simulink model "sampleModel7126_pp"  (R2018a)
settings: Solver=VariableStepAuto  StartTime=0.0  StopTime=10.0  RelTol=1e-3
undefined symbols (not defined in the file or in its folder): DiscIntNeverNeededParam
libraries: simulink x367
(part 4 of 8)

== system sampleModel7126_pp/cfblk275 ==
  cfblk1 : Inport
  Action Port : ActionPort  ActionType=then
  cfblk10 : Subsystem  TreatAsAtomicUnit=on
  cfblk11 : Subsystem  TreatAsAtomicUnit=on
  cfblk12 : Delay
  cfblk13 : Delay
  cfblk3 : simulink/Discrete/Transfer Fcn Real Zero  ZeroZ=0.75  ICPrevInput=0.0  DoSatur=off
      settings: SourceProductName=Simulink  SourceProductBaseCode=SL
  cfblk4 : simulink/Discrete/Transfer Fcn Real Zero  ZeroZ=0.75  ICPrevInput=0.0  DoSatur=off
      settings: SourceProductName=Simulink  SourceProductBaseCode=SL
  cfblk5 : simulink/Continuous/PID Controller  Controller=PID  TimeDomain=Discrete-time  SampleTime=-1  IntegratorMethod=Forward Euler  FilterMethod=Forward Euler  Form=Parallel  UseFilter=on  ControllerParametersSource=internal  P=1  I=1  D=0  N=100  InitialConditionSource=internal  InitialConditionForIntegrator=0  InitialConditionForFilter=0  ExternalReset=none  LimitOutput=off  UpperSaturationLimit=inf  LowerSaturationLimit=-inf  LinearizeAsGain=off  AntiWindupMode=none  Kb=1  TrackingMode=off  Kt=1  PParamMin=[]  PParamMax=[]  IParamMin=[]  IParamMax=[]  DParamMin=[]  DParamMax=[]  NParamMin=[]  NParamMax=[]  KbParamMin=[]  KbParamMax=[]  KtParamMin=[]  KtParamMax=[]  POutMin=[]  POutMax=[]  IOutMin=[]  IOutMax=[]  DOutMin=[]  DOutMax=[]  NOutMin=[]  NOutMax=[]  KbOutMin=[]  KbOutMax=[]  KtOutMin=[]  KtOutMax=[]  IntegratorOutMin=[]  IntegratorOutMax=[]  FilterOutMin=[]  FilterOutMax=[]  SumOutMin=[]  SumOutMax=[]  SumI1OutMin=[]  SumI1OutMax=[]  SumI2OutMin=[]  SumI2OutMax=[]  SumI3OutMin=[]  SumI3OutMax=[]  SumDOutMin=[]  SumDOutMax=[]  SaturationOutMin=[]  SaturationOutMax=[]  IntegratorContinuousStateAttributes=''  IntegratorStateMustResolveToSignalObject=off  IntegratorRTWStateStorageClass=Auto  FilterContinuousStateAttributes=''  FilterStateMustResolveToSignalObject=off  FilterRTWStateStorageClass=Auto  DifferentiatorICPrevScaledInput=0  DifferentiatorOutMin=[]  DifferentiatorOutMax=[]  FilterDiffOutCoefMin=[]  FilterDiffOutCoefMax=[]  SumDenOutMin=[]  SumDenOutMax=[]  SumNumOutMin=[]  SumNumOutMax=[]  ReciprocalOutMin=[]  ReciprocalOutMax=[]  DivideOutMin=[]  DivideOutMax=[]  TunerSelectOption=Transfer Function Based (PID Tuner App)
  cfblk6 : simulink/Discrete/Difference  ICPrevInput=0.0  OutMin=[]  OutMax=[]  OutDataTypeStr=double  OutputDataTypeScalingMode=double  OutDataType=fixdt(1, 16)  OutScaling=2^-10  DoSatur=off
  cfblk7 : DiscreteStateSpace  SampleTime=-1
  cfblk8 : DiscreteIntegrator  SampleTime=-1  OutDataTypeStr=double  ICPrevOutput=DiscIntNeverNeededParam  ICPrevScaledInput=DiscIntNeverNeededParam
  cfblk9 : If  SampleTime=1
  cyemi_{764,777,792..800} (11 alike) : DataTypeConversion  OutDataTypeStr=double
  cfblk2 : Outport
  wires:
  cfblk1/1 -> cfblk2/1
  cfblk9/1 -> cfblk10/Action
  cfblk9/2 -> cfblk11/Action
  cyemi_764/1 -> cfblk10/1(cfblk1)
  cfblk11/2(cfblk15) -> cyemi_764/1
  cyemi_777/1 -> cfblk11/1(cfblk1)
  cfblk13/1 -> cyemi_777/1
  cyemi_792/1 -> cfblk12/1
  cfblk5/1 -> cyemi_792/1
  cyemi_793/1 -> cfblk13/1
  cfblk8/1 -> cyemi_793/1
  cyemi_794/1 -> cfblk3/1
  cfblk12/1 -> cyemi_794/1
  cyemi_795/1 -> cfblk4/1
  cfblk6/1 -> cyemi_795/1
  cyemi_796/1 -> cfblk5/1
  cfblk11/1(cfblk2) -> cyemi_796/1
  cyemi_797/1 -> cfblk6/1
  cfblk3/1 -> cyemi_797/1
  cyemi_798/1 -> cfblk7/1
  cfblk11/3(cfblk16) -> cyemi_798/1
  cyemi_799/1 -> cfblk8/1
  cfblk7/1 -> cyemi_799/1
  cyemi_800/1 -> cfblk9/1
  cfblk4/1 -> cyemi_800/1

== system sampleModel7126_pp/cfblk276 ==
  cfblk1 : Inport
  cfblk9 : Inport  Port=2
  cfblk10 : Inport  Port=3
  cfblk11 : Inport  Port=4
  Action Port : ActionPort  ActionType=else
  cfblk14 : Delay
  cfblk3 : simulink/Discrete/Transfer Fcn First Order  PoleZ=0.95  ICPrevOutput=0.0  DoSatur=off
      settings: SourceProductName=Simulink
  cfblk4 : UnitDelay  SampleTime=-1
  cfblk5 : DiscreteZeroPole  Poles=[0 0.5]  Gain=1  SampleTime=-1
  cfblk6 : Delay  ShowEnablePort=on
      settings: InputPortMap=u0,e6
  cfblk7 : Delay
  cfblk8 : Delay
  cyemi_{805..811} (7 alike) : DataTypeConversion  OutDataTypeStr=double
  cyemi_812 : DataTypeConversion  OutDataTypeStr=uint8
  cfblk2 : Outport
  cfblk12 : Outport  Port=2
  cfblk13 : Outport  Port=3
  wires:
  cfblk9/1 -> cfblk2/1
  cfblk11/1 -> cfblk13/1
  cfblk8/1 -> cfblk12/1
  cyemi_805/1 -> cfblk14/1
  cfblk6/1 -> cyemi_805/1
  cyemi_806/1 -> cfblk3/1
  cfblk14/1 -> cyemi_806/1
  cyemi_807/1 -> cfblk4/1
  cfblk5/1 -> cyemi_807/1
  cyemi_808/1 -> cfblk5/1
  cfblk3/1 -> cyemi_808/1
  cyemi_809/1 -> cfblk6/1
  cfblk10/1 -> cyemi_809/1
  cyemi_810/1 -> cfblk6/2
  cfblk7/1 -> cyemi_810/1
  cyemi_811/1 -> cfblk7/1
  cfblk4/1 -> cyemi_811/1
  cyemi_812/1 -> cfblk8/1
  cfblk1/1 -> cyemi_812/1

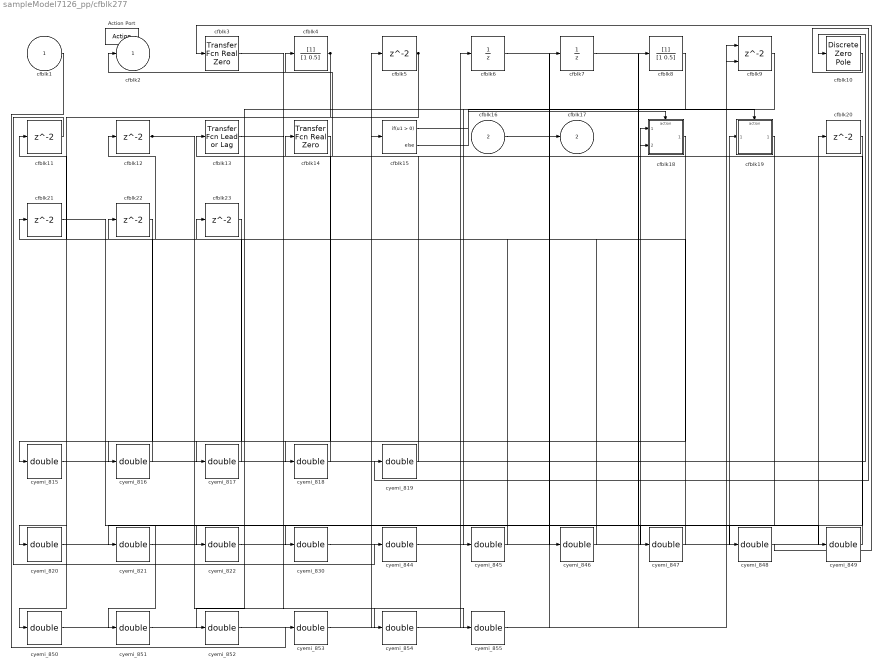
== system sampleModel7126_pp/cfblk277 ==
  cfblk1 : Inport
  cfblk16 : Inport  Port=2
  Action Port : ActionPort  ActionType=then
  cfblk10 : DiscreteZeroPole  Poles=[0 0.5]  Gain=1  SampleTime=-1
  cfblk{5,11..12,20..23} (7 alike) : Delay
  cfblk13 : simulink/Discrete/Transfer Fcn Lead or Lag  PoleZ=0.95  ZeroZ=0.75  ICPrevOutput=0.0  ICPrevInput=0.0  DoSatur=off
      settings: SourceProductName=Simulink  SourceProductBaseCode=SL
  cfblk14 : simulink/Discrete/Transfer Fcn Real Zero  ZeroZ=0.75  ICPrevInput=0.0  DoSatur=off
      settings: SourceProductName=Simulink  SourceProductBaseCode=SL
  cfblk15 : If  SampleTime=1
  cfblk18 : Subsystem  TreatAsAtomicUnit=on
  cfblk19 : Subsystem  TreatAsAtomicUnit=on
  cfblk3 : simulink/Discrete/Transfer Fcn Real Zero  ZeroZ=0.75  ICPrevInput=0.0  DoSatur=off
      settings: SourceProductName=Simulink  SourceProductBaseCode=SL
  cfblk4 : DiscreteFilter
  cfblk6 : UnitDelay  SampleTime=-1
  cfblk7 : UnitDelay  SampleTime=-1
  cfblk8 : DiscreteFilter
  cfblk9 : Delay  ShowEnablePort=on
      settings: InputPortMap=u0,e6
  cyemi_{815..822,830,844..855} (21 alike) : DataTypeConversion  OutDataTypeStr=double
  cfblk2 : Outport
  cfblk17 : Outport  Port=2
  wires:
  cfblk12/1 -> cyemi_830/1, cyemi_855/1
  cfblk5/1 -> cyemi_815/1, cyemi_817/1
  cfblk16/1 -> cfblk17/1
  cfblk4/1 -> cfblk2/1, cyemi_822/1
  cfblk15/1 -> cfblk18/Action
  cfblk15/2 -> cfblk19/Action
  cyemi_815/1 -> cfblk10/1
  cyemi_816/1 -> cfblk11/1
  cfblk18/1(cfblk2) -> cyemi_816/1
  cyemi_817/1 -> cfblk12/1
  cyemi_818/1 -> cfblk13/1
  cfblk14/1 -> cyemi_818/1
  cyemi_819/1 -> cfblk14/1
  cfblk10/1 -> cyemi_819/1
  cyemi_820/1 -> cfblk15/1
  cfblk22/1 -> cyemi_820/1
  cyemi_821/1 -> cfblk18/1(cfblk1)
  cfblk20/1 -> cyemi_821/1
  cyemi_822/1 -> cfblk18/2(cfblk8)
  cyemi_830/1 -> cfblk19/1(cfblk1)
  cyemi_844/1 -> cfblk20/1
  cfblk11/1 -> cyemi_844/1
  cyemi_845/1 -> cfblk21/1
  cfblk9/1 -> cyemi_845/1
  cyemi_846/1 -> cfblk22/1
  cfblk6/1 -> cyemi_846/1
  cyemi_847/1 -> cfblk23/1
  cfblk13/1 -> cyemi_847/1
  cyemi_848/1 -> cfblk3/1
  cfblk21/1 -> cyemi_848/1
  cyemi_849/1 -> cfblk4/1
  cfblk7/1 -> cyemi_849/1
  cyemi_850/1 -> cfblk5/1
  cfblk23/1 -> cyemi_850/1
  cyemi_851/1 -> cfblk6/1
  cfblk19/1(cfblk2) -> cyemi_851/1
  cyemi_852/1 -> cfblk7/1
  cfblk8/1 -> cyemi_852/1
  cyemi_853/1 -> cfblk8/1
  cfblk1/1 -> cyemi_853/1
  cyemi_854/1 -> cfblk9/1
  cfblk3/1 -> cyemi_854/1
  cyemi_855/1 -> cfblk9/2

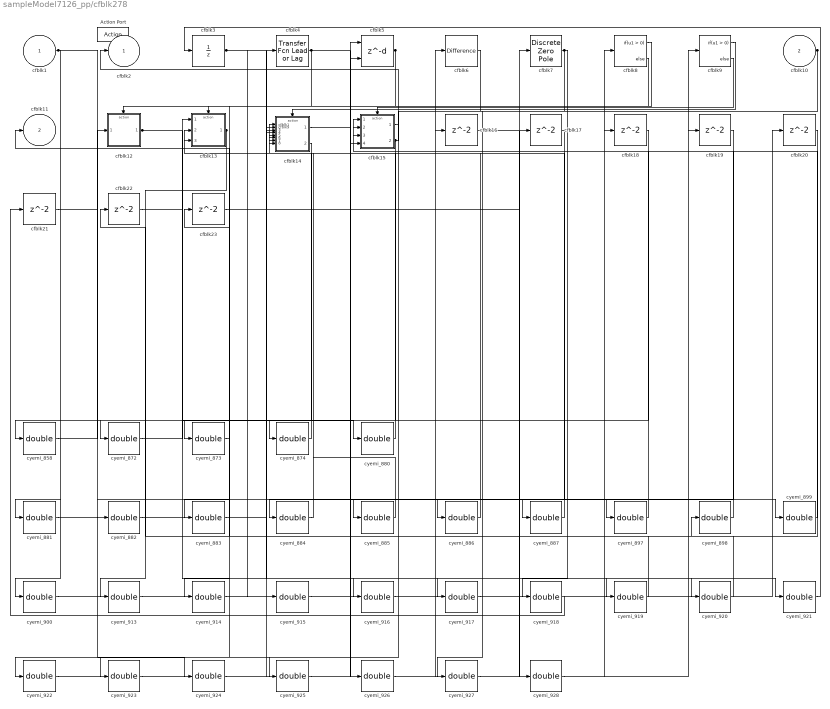
== system sampleModel7126_pp/cfblk278 ==
  cfblk1 : Inport
  cfblk10 : Inport  Port=2
  Action Port : ActionPort  ActionType=else
  cfblk12 : Subsystem  TreatAsAtomicUnit=on
  cfblk13 : Subsystem  TreatAsAtomicUnit=on
  cfblk14 : Subsystem  TreatAsAtomicUnit=on
  cfblk15 : Subsystem  TreatAsAtomicUnit=on
  cfblk{16..23} (8 alike) : Delay
  cfblk3 : UnitDelay  SampleTime=-1
  cfblk4 : simulink/Discrete/Transfer Fcn Lead or Lag  PoleZ=0.95  ZeroZ=0.75  ICPrevOutput=0.0  ICPrevInput=0.0  DoSatur=off
      settings: SourceProductName=Simulink  SourceProductBaseCode=SL
  cfblk5 : Delay  DelayLengthSource=Input port
      settings: InputPortMap=u0,p1
  cfblk6 : simulink/Discrete/Difference  ICPrevInput=0.0  OutMin=[]  OutMax=[]  OutDataTypeStr=double  OutputDataTypeScalingMode=double  OutDataType=fixdt(1, 16)  OutScaling=2^-10  DoSatur=off
  cfblk7 : DiscreteZeroPole  Poles=[0 0.5]  Gain=1  SampleTime=-1
  cfblk8 : If  SampleTime=1
  cfblk9 : If  SampleTime=1
  cyemi_{858,872..874,880..887,897..900,913..928} (32 alike) : DataTypeConversion  OutDataTypeStr=double
  cfblk2 : Outport
  cfblk11 : Outport  Port=2
  wires:
  cfblk5/1 -> cyemi_872/1, cyemi_914/1
  cfblk13/1(cfblk2) -> cfblk11/1, cyemi_913/1
  cfblk12/1(cfblk2) -> cyemi_917/1, cyemi_921/1
  cfblk1/1 -> cyemi_881/1, cyemi_897/1, cyemi_900/1, cyemi_924/1
  cfblk7/1 -> cyemi_918/1, cyemi_927/1
  cfblk4/1 -> cyemi_919/1, cyemi_920/1, cyemi_923/1
  cfblk3/1 -> cyemi_915/1, cyemi_916/1
  cfblk10/1 -> cyemi_886/1, cyemi_925/1
  cfblk15/2(cfblk16) -> cfblk2/1, cyemi_883/1, cyemi_885/1
  cfblk8/1 -> cfblk12/Action
  cfblk8/2 -> cfblk13/Action
  cfblk9/1 -> cfblk14/Action
  cfblk9/2 -> cfblk15/Action
  cyemi_858/1 -> cfblk12/1(cfblk1)
  cfblk14/2(cfblk16) -> cyemi_858/1
  cyemi_872/1 -> cfblk13/1(cfblk1)
  cyemi_873/1 -> cfblk13/2(cfblk8)
  cfblk6/1 -> cyemi_873/1
  cyemi_874/1 -> cfblk13/3(cfblk9)
  cfblk18/1 -> cyemi_874/1
  cyemi_880/1 -> cfblk14/1(cfblk1)
  cfblk22/1 -> cyemi_880/1
  cyemi_881/1 -> cfblk14/2(cfblk9)
  cyemi_882/1 -> cfblk14/3(cfblk10)
  cfblk21/1 -> cyemi_882/1
  cyemi_883/1 -> cfblk14/4(cfblk11)
  cyemi_884/1 -> cfblk14/5(cfblk12)
  cfblk17/1 -> cyemi_884/1
  cyemi_885/1 -> cfblk14/6(cfblk13)
  cyemi_886/1 -> cfblk14/7(cfblk14)
  cyemi_887/1 -> cfblk14/8(cfblk15)
  cfblk19/1 -> cyemi_887/1
  cyemi_897/1 -> cfblk15/1(cfblk1)
  cyemi_898/1 -> cfblk15/2(cfblk13)
  cfblk20/1 -> cyemi_898/1
  cyemi_899/1 -> cfblk15/3(cfblk14)
  cfblk16/1 -> cyemi_899/1
  cyemi_900/1 -> cfblk15/4(cfblk15)
  cyemi_913/1 -> cfblk16/1
  cyemi_914/1 -> cfblk17/1
  cyemi_915/1 -> cfblk18/1
  cyemi_916/1 -> cfblk19/1
  cyemi_917/1 -> cfblk20/1
  cyemi_918/1 -> cfblk21/1
  cyemi_919/1 -> cfblk22/1
  cyemi_920/1 -> cfblk23/1
  cyemi_921/1 -> cfblk3/1
  cyemi_922/1 -> cfblk4/1
  cfblk15/1(cfblk2) -> cyemi_922/1
  cyemi_923/1 -> cfblk5/1
  cyemi_924/1 -> cfblk5/2
  cyemi_925/1 -> cfblk6/1
  cyemi_926/1 -> cfblk7/1
  cfblk14/1(cfblk2) -> cyemi_926/1
  cyemi_927/1 -> cfblk8/1
  cyemi_928/1 -> cfblk9/1
  cfblk23/1 -> cyemi_928/1

== system sampleModel7126_pp/cfblk279 ==
  cfblk1 : Inport
  cfblk8 : Inport  Port=2
  Action Port : ActionPort  ActionType=then
  cfblk10 : Delay
  cfblk11 : Delay
  cfblk3 : simulink/Discrete/Transfer Fcn First Order  PoleZ=0.95  ICPrevOutput=0.0  DoSatur=off
      settings: SourceProductName=Simulink
  cfblk4 : simulink/Discrete/Tapped Delay  vinit=0.0  samptime=-1  NumDelays=1  DelayOrder=Oldest  includeCurrent=off
  cfblk5 : DiscreteTransferFcn
  cfblk6 : DiscreteStateSpace  SampleTime=-1
  cfblk7 : Delay  ShowEnablePort=on
      settings: InputPortMap=u0,e6
  cyemi_{931..938} (8 alike) : DataTypeConversion  OutDataTypeStr=double
  cfblk2 : Outport
  cfblk9 : Outport  Port=2
  wires:
  cfblk1/1 -> cfblk9/1
  cfblk5/1 -> cfblk2/1, cyemi_931/1
  cyemi_931/1 -> cfblk10/1
  cyemi_932/1 -> cfblk11/1
  cfblk6/1 -> cyemi_932/1
  cyemi_933/1 -> cfblk3/1
  cfblk8/1 -> cyemi_933/1
  cyemi_934/1 -> cfblk4/1
  cfblk11/1 -> cyemi_934/1
  cyemi_935/1 -> cfblk5/1
  cfblk7/1 -> cyemi_935/1
  cyemi_936/1 -> cfblk6/1
  cfblk4/1 -> cyemi_936/1
  cyemi_937/1 -> cfblk7/1
  cfblk3/1 -> cyemi_937/1
  cyemi_938/1 -> cfblk7/2
  cfblk10/1 -> cyemi_938/1

== system sampleModel7126_pp/cfblk280 ==
  cfblk1 : Inport
  cfblk10 : Inport  Port=2
  Action Port : ActionPort  ActionType=else
  cfblk13 : Subsystem  TreatAsAtomicUnit=on
  cfblk14 : Subsystem  TreatAsAtomicUnit=on
  cfblk15 : Delay
  cfblk16 : Delay
  cfblk3 : Delay  DelayLengthSource=Input port
      settings: InputPortMap=u0,p1
  cfblk4 : simulink/Discrete/Transfer Fcn Lead or Lag  PoleZ=0.95  ZeroZ=0.75  ICPrevOutput=0.0  ICPrevInput=0.0  DoSatur=off
      settings: SourceProductName=Simulink  SourceProductBaseCode=SL
  cfblk5 : simulink/Discrete/Transfer Fcn First Order  PoleZ=0.95  ICPrevOutput=0.0  DoSatur=off
      settings: SourceProductName=Simulink
  cfblk6 : simulink/Discrete/Tapped Delay  vinit=0.0  samptime=-1  NumDelays=1  DelayOrder=Oldest  includeCurrent=off
  cfblk7 : simulink/Discrete/Transfer Fcn Lead or Lag  PoleZ=0.95  ZeroZ=0.75  ICPrevOutput=0.0  ICPrevInput=0.0  DoSatur=off
      settings: SourceProductName=Simulink  SourceProductBaseCode=SL
  cfblk8 : Delay  ShowEnablePort=on
      settings: InputPortMap=u0,e6
  cfblk9 : If  SampleTime=1
  cyemi_{942,961,963,965,969..970} (6 alike) : DataTypeConversion  OutDataTypeStr=double
  cyemi_{951,953,966..968} (5 alike) : DataTypeConversion  OutDataTypeStr=uint8
  cyemi_952 : DataTypeConversion  OutDataTypeStr=fixdt('ufix8_E6')
  cyemi_960 : DataTypeConversion  OutDataTypeStr=fixdt('ufix8_E6')
  cyemi_962 : DataTypeConversion  OutDataTypeStr=fixdt('ufix8_E3')
  cyemi_964 : DataTypeConversion  OutDataTypeStr=fixdt('ufix8_E3')
  cfblk2 : Outport
  cfblk11 : Outport  Port=2
  cfblk12 : Outport  Port=3
  wires:
  cfblk1/1 -> cfblk11/1, cyemi_953/1, cyemi_966/1
  cfblk10/1 -> cyemi_942/1, cyemi_969/1
  cfblk7/1 -> cfblk12/1, cyemi_962/1
  cfblk14/2(cfblk10) -> cfblk2/1
  cfblk9/1 -> cfblk13/Action
  cfblk9/2 -> cfblk14/Action
  cyemi_942/1 -> cfblk13/1(cfblk1)
  cyemi_951/1 -> cfblk14/1(cfblk1)
  cfblk6/1 -> cyemi_951/1
  cyemi_952/1 -> cfblk14/2(cfblk8)
  cfblk15/1 -> cyemi_952/1
  cyemi_953/1 -> cfblk14/3(cfblk9)
  cyemi_960/1 -> cfblk15/1
  cfblk4/1 -> cyemi_960/1
  cyemi_961/1 -> cfblk16/1
  cfblk13/2(cfblk8) -> cyemi_961/1
  cyemi_962/1 -> cfblk3/1
  cyemi_963/1 -> cfblk3/2
  cfblk5/1 -> cyemi_963/1
  cyemi_964/1 -> cfblk4/1
  cfblk3/1 -> cyemi_964/1
  cyemi_965/1 -> cfblk5/1
  cfblk13/1(cfblk2) -> cyemi_965/1
  cyemi_966/1 -> cfblk6/1
  cyemi_967/1 -> cfblk7/1
  cfblk8/1 -> cyemi_967/1
  cyemi_968/1 -> cfblk8/1
  cfblk14/1(cfblk2) -> cyemi_968/1
  cyemi_969/1 -> cfblk8/2
  cyemi_970/1 -> cfblk9/1
  cfblk16/1 -> cyemi_970/1

== system sampleModel7126_pp/cfblk281 ==
  cfblk1 : Inport
  cfblk12 : Inport  Port=2
  cfblk13 : Inport  Port=3
  Action Port : ActionPort  ActionType=then
  cfblk10 : Delay
  cfblk11 : simulink/Discrete/Transfer Fcn First Order  PoleZ=0.95  ICPrevOutput=0.0  DoSatur=off
      settings: SourceProductName=Simulink
  cfblk3 : simulink/Discrete/Transfer Fcn Real Zero  ZeroZ=0.75  ICPrevInput=0.0  DoSatur=off
      settings: SourceProductName=Simulink  SourceProductBaseCode=SL
  cfblk4 : simulink/Continuous/PID Controller  Controller=PID  TimeDomain=Discrete-time  SampleTime=-1  IntegratorMethod=Forward Euler  FilterMethod=Forward Euler  Form=Parallel  UseFilter=on  ControllerParametersSource=internal  P=1  I=1  D=0  N=100  InitialConditionSource=internal  InitialConditionForIntegrator=0  InitialConditionForFilter=0  ExternalReset=none  LimitOutput=off  UpperSaturationLimit=inf  LowerSaturationLimit=-inf  LinearizeAsGain=off  AntiWindupMode=none  Kb=1  TrackingMode=off  Kt=1  PParamMin=[]  PParamMax=[]  IParamMin=[]  IParamMax=[]  DParamMin=[]  DParamMax=[]  NParamMin=[]  NParamMax=[]  KbParamMin=[]  KbParamMax=[]  KtParamMin=[]  KtParamMax=[]  POutMin=[]  POutMax=[]  IOutMin=[]  IOutMax=[]  DOutMin=[]  DOutMax=[]  NOutMin=[]  NOutMax=[]  KbOutMin=[]  KbOutMax=[]  KtOutMin=[]  KtOutMax=[]  IntegratorOutMin=[]  IntegratorOutMax=[]  FilterOutMin=[]  FilterOutMax=[]  SumOutMin=[]  SumOutMax=[]  SumI1OutMin=[]  SumI1OutMax=[]  SumI2OutMin=[]  SumI2OutMax=[]  SumI3OutMin=[]  SumI3OutMax=[]  SumDOutMin=[]  SumDOutMax=[]  SaturationOutMin=[]  SaturationOutMax=[]  IntegratorContinuousStateAttributes=''  IntegratorStateMustResolveToSignalObject=off  IntegratorRTWStateStorageClass=Auto  FilterContinuousStateAttributes=''  FilterStateMustResolveToSignalObject=off  FilterRTWStateStorageClass=Auto  DifferentiatorICPrevScaledInput=0  DifferentiatorOutMin=[]  DifferentiatorOutMax=[]  FilterDiffOutCoefMin=[]  FilterDiffOutCoefMax=[]  SumDenOutMin=[]  SumDenOutMax=[]  SumNumOutMin=[]  SumNumOutMax=[]  ReciprocalOutMin=[]  ReciprocalOutMax=[]  DivideOutMin=[]  DivideOutMax=[]  TunerSelectOption=Transfer Function Based (PID Tuner App)
  cfblk5 : Delay  ShowEnablePort=on
      settings: InputPortMap=u0,e6
  cfblk6 : Delay
  cfblk7 : Delay  DelayLengthSource=Input port
      settings: InputPortMap=u0,p1
  cfblk8 : DiscreteStateSpace  SampleTime=-1
  cfblk9 : DiscreteFilter
  cyemi_{974..984} (11 alike) : DataTypeConversion  OutDataTypeStr=double
  cfblk2 : Outport
  wires:
  cfblk7/1 -> cfblk2/1
  cyemi_974/1 -> cfblk10/1
  cfblk5/1 -> cyemi_974/1
  cyemi_975/1 -> cfblk11/1
  cfblk8/1 -> cyemi_975/1
  cyemi_976/1 -> cfblk3/1
  cfblk4/1 -> cyemi_976/1
  cyemi_977/1 -> cfblk4/1
  cfblk6/1 -> cyemi_977/1
  cyemi_978/1 -> cfblk5/1
  cfblk9/1 -> cyemi_978/1
  cyemi_979/1 -> cfblk5/2
  cfblk11/1 -> cyemi_979/1
  cyemi_980/1 -> cfblk6/1
  cfblk1/1 -> cyemi_980/1
  cyemi_981/1 -> cfblk7/1
  cfblk12/1 -> cyemi_981/1
  cyemi_982/1 -> cfblk7/2
  cfblk10/1 -> cyemi_982/1
  cyemi_983/1 -> cfblk8/1
  cfblk13/1 -> cyemi_983/1
  cyemi_984/1 -> cfblk9/1
  cfblk3/1 -> cyemi_984/1

== system sampleModel7126_pp/cfblk282 ==
  cfblk1 : Inport
  cfblk10 : Inport  Port=2
  cfblk11 : Inport  Port=3
  Action Port : ActionPort  ActionType=else
  cfblk16 : Delay
  cfblk17 : Delay
  cfblk3 : simulink/Discrete/Tapped Delay  vinit=0.0  samptime=-1  NumDelays=1  DelayOrder=Oldest  includeCurrent=off
  cfblk4 : DiscreteIntegrator  SampleTime=-1  OutDataTypeStr=double  ICPrevOutput=DiscIntNeverNeededParam  ICPrevScaledInput=DiscIntNeverNeededParam
  cfblk5 : Delay  ShowEnablePort=on
      settings: InputPortMap=u0,e6
  cfblk6 : simulink/Discrete/Tapped Delay  vinit=0.0  samptime=-1  NumDelays=1  DelayOrder=Oldest  includeCurrent=off
  cfblk7 : simulink/Discrete/Tapped Delay  vinit=0.0  samptime=-1  NumDelays=1  DelayOrder=Oldest  includeCurrent=off
  cfblk8 : Delay  DelayLengthSource=Input port
      settings: InputPortMap=u0,p1
  cfblk9 : DiscreteFir
  cyemi_{988..998} (11 alike) : DataTypeConversion  OutDataTypeStr=double
  cfblk2 : Outport
  cfblk12 : Outport  Port=2
  cfblk13 : Outport  Port=3
  cfblk14 : Outport  Port=4
  cfblk15 : Outport  Port=5
  wires:
  cfblk8/1 -> cfblk15/1, cfblk12/1, cyemi_991/1, cyemi_995/1
  cfblk4/1 -> cfblk14/1
  cfblk11/1 -> cfblk2/1, cfblk13/1
  cyemi_988/1 -> cfblk16/1
  cfblk7/1 -> cyemi_988/1
  cyemi_989/1 -> cfblk17/1
  cfblk9/1 -> cyemi_989/1
  cyemi_990/1 -> cfblk3/1
  cfblk5/1 -> cyemi_990/1
  cyemi_991/1 -> cfblk4/1
  cyemi_992/1 -> cfblk5/1
  cfblk16/1 -> cyemi_992/1
  cyemi_993/1 -> cfblk5/2
  cfblk1/1 -> cyemi_993/1
  cyemi_994/1 -> cfblk6/1
  cfblk17/1 -> cyemi_994/1
  cyemi_995/1 -> cfblk7/1
  cyemi_996/1 -> cfblk8/1
  cfblk3/1 -> cyemi_996/1
  cyemi_997/1 -> cfblk8/2
  cfblk10/1 -> cyemi_997/1
  cyemi_998/1 -> cfblk9/1
  cfblk6/1 -> cyemi_998/1

== system sampleModel7126_pp/cfblk283 ==
  cfblk1 : Inport
  cfblk14 : Inport  Port=2
  Action Port : ActionPort  ActionType=then
  cfblk10 : DiscreteTransferFcn
  cfblk11 : DiscreteZeroPole  Poles=[0 0.5]  Gain=1  SampleTime=-1
  cfblk12 : DiscreteFir
  cfblk13 : Delay  DelayLengthSource=Input port
      settings: InputPortMap=u0,p1
  cfblk3 : simulink/Discrete/Difference  ICPrevInput=0.0  OutMin=[]  OutMax=[]  OutDataTypeStr=double  OutputDataTypeScalingMode=double  OutDataType=fixdt(1, 16)  OutScaling=2^-10  DoSatur=off
  cfblk4 : simulink/Discrete/Transfer Fcn Real Zero  ZeroZ=0.75  ICPrevInput=0.0  DoSatur=off
      settings: SourceProductName=Simulink  SourceProductBaseCode=SL
  cfblk5 : simulink/Discrete/Transfer Fcn Lead or Lag  PoleZ=0.95  ZeroZ=0.75  ICPrevOutput=0.0  ICPrevInput=0.0  DoSatur=off
      settings: SourceProductName=Simulink  SourceProductBaseCode=SL
  cfblk6 : simulink/Discrete/Difference  ICPrevInput=0.0  OutMin=[]  OutMax=[]  OutDataTypeStr=double  OutputDataTypeScalingMode=double  OutDataType=fixdt(1, 16)  OutScaling=2^-10  DoSatur=off
  cfblk7 : simulink/Discrete/Tapped Delay  vinit=0.0  samptime=-1  NumDelays=1  DelayOrder=Oldest  includeCurrent=off
  cfblk8 : simulink/Continuous/PID Controller  Controller=PID  TimeDomain=Discrete-time  SampleTime=-1  IntegratorMethod=Forward Euler  FilterMethod=Forward Euler  Form=Parallel  UseFilter=on  ControllerParametersSource=internal  P=1  I=1  D=0  N=100  InitialConditionSource=internal  InitialConditionForIntegrator=0  InitialConditionForFilter=0  ExternalReset=none  LimitOutput=off  UpperSaturationLimit=inf  LowerSaturationLimit=-inf  LinearizeAsGain=off  AntiWindupMode=none  Kb=1  TrackingMode=off  Kt=1  PParamMin=[]  PParamMax=[]  IParamMin=[]  IParamMax=[]  DParamMin=[]  DParamMax=[]  NParamMin=[]  NParamMax=[]  KbParamMin=[]  KbParamMax=[]  KtParamMin=[]  KtParamMax=[]  POutMin=[]  POutMax=[]  IOutMin=[]  IOutMax=[]  DOutMin=[]  DOutMax=[]  NOutMin=[]  NOutMax=[]  KbOutMin=[]  KbOutMax=[]  KtOutMin=[]  KtOutMax=[]  IntegratorOutMin=[]  IntegratorOutMax=[]  FilterOutMin=[]  FilterOutMax=[]  SumOutMin=[]  SumOutMax=[]  SumI1OutMin=[]  SumI1OutMax=[]  SumI2OutMin=[]  SumI2OutMax=[]  SumI3OutMin=[]  SumI3OutMax=[]  SumDOutMin=[]  SumDOutMax=[]  SaturationOutMin=[]  SaturationOutMax=[]  IntegratorContinuousStateAttributes=''  IntegratorStateMustResolveToSignalObject=off  IntegratorRTWStateStorageClass=Auto  FilterContinuousStateAttributes=''  FilterStateMustResolveToSignalObject=off  FilterRTWStateStorageClass=Auto  DifferentiatorICPrevScaledInput=0  DifferentiatorOutMin=[]  DifferentiatorOutMax=[]  FilterDiffOutCoefMin=[]  FilterDiffOutCoefMax=[]  SumDenOutMin=[]  SumDenOutMax=[]  SumNumOutMin=[]  SumNumOutMax=[]  ReciprocalOutMin=[]  ReciprocalOutMax=[]  DivideOutMin=[]  DivideOutMax=[]  TunerSelectOption=Transfer Function Based (PID Tuner App)
  cfblk9 : simulink/Discrete/Transfer Fcn Lead or Lag  PoleZ=0.95  ZeroZ=0.75  ICPrevOutput=0.0  ICPrevInput=0.0  DoSatur=off
      settings: SourceProductName=Simulink  SourceProductBaseCode=SL
  cyemi_{1001..1012} (12 alike) : DataTypeConversion  OutDataTypeStr=double
  cfblk2 : Outport
  cfblk15 : Outport  Port=2
  cfblk16 : Outport  Port=3
  cfblk17 : Outport  Port=4
  wires:
  cfblk14/1 -> cfblk2/1, cyemi_1012/1
  cfblk10/1 -> cfblk17/1, cyemi_1005/1
  cfblk9/1 -> cfblk16/1
  cfblk8/1 -> cyemi_1001/1, cyemi_1002/1
  cfblk4/1 -> cfblk15/1
  cyemi_1001/1 -> cfblk10/1
  cyemi_1002/1 -> cfblk11/1
  cyemi_1003/1 -> cfblk12/1
  cfblk13/1 -> cyemi_1003/1
  cyemi_1004/1 -> cfblk13/1
  cfblk3/1 -> cyemi_1004/1
  cyemi_1005/1 -> cfblk13/2
  cyemi_1006/1 -> cfblk3/1
  cfblk11/1 -> cyemi_1006/1
  cyemi_1007/1 -> cfblk4/1
  cfblk5/1 -> cyemi_1007/1
  cyemi_1008/1 -> cfblk5/1
  cfblk6/1 -> cyemi_1008/1
  cyemi_1009/1 -> cfblk6/1
  cfblk12/1 -> cyemi_1009/1
  cyemi_1010/1 -> cfblk7/1
  cfblk1/1 -> cyemi_1010/1
  cyemi_1011/1 -> cfblk8/1
  cfblk7/1 -> cyemi_1011/1
  cyemi_1012/1 -> cfblk9/1

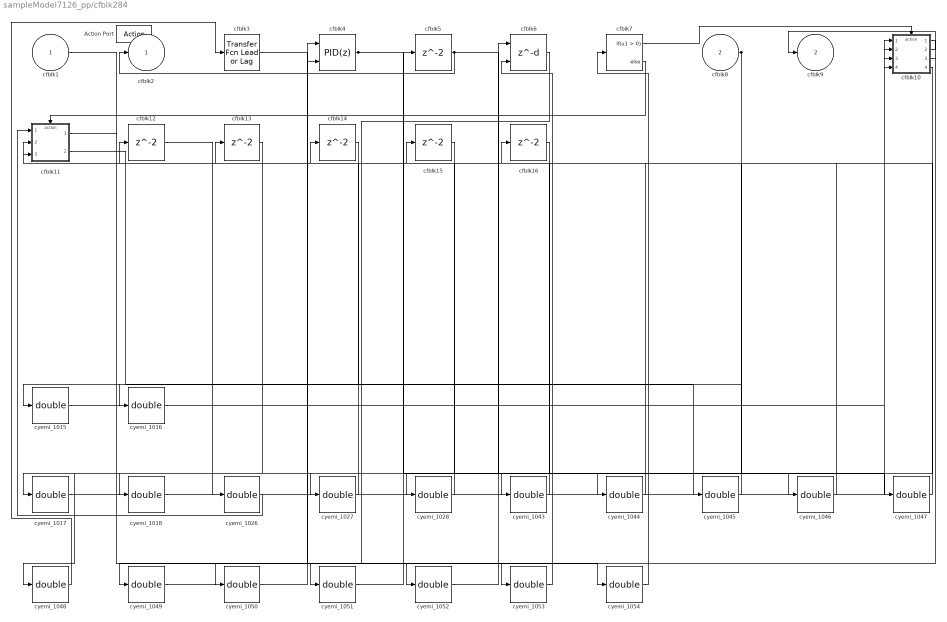
== system sampleModel7126_pp/cfblk284 ==
  cfblk1 : Inport
  cfblk8 : Inport  Port=2
  Action Port : ActionPort  ActionType=else
  cfblk10 : Subsystem  TreatAsAtomicUnit=on
  cfblk11 : Subsystem  TreatAsAtomicUnit=on
  cfblk{5,12..16} (6 alike) : Delay
  cfblk3 : simulink/Discrete/Transfer Fcn Lead or Lag  PoleZ=0.95  ZeroZ=0.75  ICPrevOutput=0.0  ICPrevInput=0.0  DoSatur=off
      settings: SourceProductName=Simulink  SourceProductBaseCode=SL
  cfblk4 : simulink/Continuous/PID Controller (2DOF)  Controller=PID  TimeDomain=Discrete-time  SampleTime=-1  IntegratorMethod=Forward Euler  FilterMethod=Forward Euler  Form=Parallel  UseFilter=on  ControllerParametersSource=internal  P=1  I=1  D=0  N=100  b=1  c=1  InitialConditionSource=internal  InitialConditionForIntegrator=0  InitialConditionForFilter=0  ExternalReset=none  LimitOutput=off  UpperSaturationLimit=inf  LowerSaturationLimit=-inf  LinearizeAsGain=off  AntiWindupMode=none  Kb=1  TrackingMode=off  Kt=1  PParamMin=[]  PParamMax=[]  IParamMin=[]  IParamMax=[]  DParamMin=[]  DParamMax=[]  NParamMin=[]  NParamMax=[]  bParamMin=[]  bParamMax=[]  cParamMin=[]  cParamMax=[]  KbParamMin=[]  KbParamMax=[]  KtParamMin=[]  KtParamMax=[]  POutMin=[]  POutMax=[]  IOutMin=[]  IOutMax=[]  DOutMin=[]  DOutMax=[]  NOutMin=[]  NOutMax=[]  bOutMin=[]  bOutMax=[]  cOutMin=[]  cOutMax=[]  KbOutMin=[]  KbOutMax=[]  KtOutMin=[]  KtOutMax=[]  IntegratorOutMin=[]  IntegratorOutMax=[]  FilterOutMin=[]  FilterOutMax=[]  SumOutMin=[]  SumOutMax=[]  Sum1OutMin=[]  Sum1OutMax=[]  Sum2OutMin=[]  Sum2OutMax=[]  Sum3OutMin=[]  Sum3OutMax=[]  SumI1OutMin=[]  SumI1OutMax=[]  SumI2OutMin=[]  SumI2OutMax=[]  SumI3OutMin=[]  SumI3OutMax=[]  SumDOutMin=[]  SumDOutMax=[]  SaturationOutMin=[]  SaturationOutMax=[]  IntegratorContinuousStateAttributes=''  IntegratorStateMustResolveToSignalObject=off  IntegratorRTWStateStorageClass=Auto  FilterContinuousStateAttributes=''  FilterStateMustResolveToSignalObject=off  FilterRTWStateStorageClass=Auto  DifferentiatorICPrevScaledInput=0  DifferentiatorOutMin=[]  DifferentiatorOutMax=[]  FilterDiffOutCoefMin=[]  FilterDiffOutCoefMax=[]  SumDenOutMin=[]  SumDenOutMax=[]  SumNumOutMin=[]  SumNumOutMax=[]  ReciprocalOutMin=[]  ReciprocalOutMax=[]  DivideOutMin=[]  DivideOutMax=[]  TunerSelectOption=Transfer Function Based (PID Tuner App)
  cfblk6 : Delay  DelayLengthSource=Input port
      settings: InputPortMap=u0,p1
  cfblk7 : If  SampleTime=1
  cyemi_{1015..1018,1026..1028,1043..1054} (19 alike) : DataTypeConversion  OutDataTypeStr=double
  cfblk2 : Outport
  cfblk9 : Outport  Port=2
  wires:
  cfblk8/1 -> cyemi_1016/1, cyemi_1048/1
  cfblk5/1 -> cfblk2/1, cyemi_1044/1
  cfblk4/1 -> cyemi_1043/1, cyemi_1046/1, cyemi_1047/1
  cfblk10/2(cfblk13) -> cfblk9/1
  cfblk7/1 -> cfblk10/Action
  cfblk7/2 -> cfblk11/Action
  cyemi_1015/1 -> cfblk10/1(cfblk1)
  cfblk14/1 -> cyemi_1015/1
  cyemi_1016/1 -> cfblk10/2(cfblk10)
  cyemi_1017/1 -> cfblk10/3(cfblk11)
  cfblk16/1 -> cyemi_1017/1
  cyemi_1018/1 -> cfblk10/4(cfblk12)
  cfblk13/1 -> cyemi_1018/1
  cyemi_1026/1 -> cfblk11/1(cfblk1)
  cfblk12/1 -> cyemi_1026/1
  cyemi_1027/1 -> cfblk11/2(cfblk13)
  cfblk10/4(cfblk15) -> cyemi_1027/1
  cyemi_1028/1 -> cfblk11/3(cfblk14)
  cfblk15/1 -> cyemi_1028/1
  cyemi_1043/1 -> cfblk12/1
  cyemi_1044/1 -> cfblk13/1
  cyemi_1045/1 -> cfblk14/1
  cfblk11/2(cfblk15) -> cyemi_1045/1
  cyemi_1046/1 -> cfblk15/1
  cyemi_1047/1 -> cfblk16/1
  cyemi_1048/1 -> cfblk3/1
  cyemi_1049/1 -> cfblk4/1
  cfblk10/1(cfblk2) -> cyemi_1049/1
  cyemi_1050/1 -> cfblk4/2
  cfblk10/3(cfblk14) -> cyemi_1050/1
  cyemi_1051/1 -> cfblk5/1
  cfblk6/1 -> cyemi_1051/1
  cyemi_1052/1 -> cfblk6/1
  cfblk3/1 -> cyemi_1052/1
  cyemi_1053/1 -> cfblk6/2
  cfblk11/1(cfblk2) -> cyemi_1053/1
  cyemi_1054/1 -> cfblk7/1
  cfblk1/1 -> cyemi_1054/1

== system sampleModel7126_pp/cfblk285 ==
  cfblk1 : Inport
  cfblk8 : Inport  Port=2
  cfblk9 : Inport  Port=3
  Action Port : ActionPort  ActionType=then
  cfblk3 : DiscreteZeroPole  Poles=[0 0.5]  Gain=1  SampleTime=-1
  cfblk4 : simulink/Discrete/Tapped Delay  vinit=0.0  samptime=-1  NumDelays=1  DelayOrder=Oldest  includeCurrent=off
  cfblk5 : simulink/Discrete/Transfer Fcn Lead or Lag  PoleZ=0.95  ZeroZ=0.75  ICPrevOutput=0.0  ICPrevInput=0.0  DoSatur=off
      settings: SourceProductName=Simulink  SourceProductBaseCode=SL
  cfblk6 : DiscreteZeroPole  Poles=[0 0.5]  Gain=1  SampleTime=-1
  cfblk7 : DiscreteTransferFcn
  cyemi_{1058..1062} (5 alike) : DataTypeConversion  OutDataTypeStr=double
  cfblk2 : Outport
  wires:
  cfblk3/1 -> cfblk2/1
  cyemi_1058/1 -> cfblk3/1
  cfblk6/1 -> cyemi_1058/1
  cyemi_1059/1 -> cfblk4/1
  cfblk7/1 -> cyemi_1059/1
  cyemi_1060/1 -> cfblk5/1
  cfblk1/1 -> cyemi_1060/1
  cyemi_1061/1 -> cfblk6/1
  cfblk9/1 -> cyemi_1061/1
  cyemi_1062/1 -> cfblk7/1
  cfblk5/1 -> cyemi_1062/1

== system sampleModel7126_pp/cfblk286 ==
  cfblk1 : Inport
  cfblk7 : Inport  Port=2
  cfblk8 : Inport  Port=3
  Action Port : ActionPort  ActionType=else
  cfblk3 : simulink/Discrete/Difference  ICPrevInput=0.0  OutMin=[]  OutMax=[]  OutDataTypeStr=double  OutputDataTypeScalingMode=double  OutDataType=fixdt(1, 16)  OutScaling=2^-10  DoSatur=off
  cfblk4 : UnitDelay  SampleTime=-1
  cfblk5 : UnitDelay  SampleTime=-1
  cfblk6 : DiscreteStateSpace  SampleTime=-1
  cyemi_1066 : DataTypeConversion  OutDataTypeStr=double
  cyemi_1067 : DataTypeConversion  OutDataTypeStr=uint8
  cyemi_1068 : DataTypeConversion  OutDataTypeStr=double
  cyemi_1069 : DataTypeConversion  OutDataTypeStr=double
  cfblk2 : Outport
  wires:
  cfblk4/1 -> cfblk2/1
  cyemi_1066/1 -> cfblk3/1
  cfblk5/1 -> cyemi_1066/1
  cyemi_1067/1 -> cfblk4/1
  cfblk1/1 -> cyemi_1067/1
  cyemi_1068/1 -> cfblk5/1
  cfblk8/1 -> cyemi_1068/1
  cyemi_1069/1 -> cfblk6/1
  cfblk7/1 -> cyemi_1069/1

== system sampleModel7126_pp/cfblk287 ==
  cfblk1 : Inport
  cfblk8 : Inport  Port=2
  cfblk9 : Inport  Port=3
  Action Port : ActionPort  ActionType=then
  cfblk10 : Delay
  cfblk3 : simulink/Continuous/PID Controller (2DOF)  Controller=PID  TimeDomain=Discrete-time  SampleTime=-1  IntegratorMethod=Forward Euler  FilterMethod=Forward Euler  Form=Parallel  UseFilter=on  ControllerParametersSource=internal  P=1  I=1  D=0  N=100  b=1  c=1  InitialConditionSource=internal  InitialConditionForIntegrator=0  InitialConditionForFilter=0  ExternalReset=none  LimitOutput=off  UpperSaturationLimit=inf  LowerSaturationLimit=-inf  LinearizeAsGain=off  AntiWindupMode=none  Kb=1  TrackingMode=off  Kt=1  PParamMin=[]  PParamMax=[]  IParamMin=[]  IParamMax=[]  DParamMin=[]  DParamMax=[]  NParamMin=[]  NParamMax=[]  bParamMin=[]  bParamMax=[]  cParamMin=[]  cParamMax=[]  KbParamMin=[]  KbParamMax=[]  KtParamMin=[]  KtParamMax=[]  POutMin=[]  POutMax=[]  IOutMin=[]  IOutMax=[]  DOutMin=[]  DOutMax=[]  NOutMin=[]  NOutMax=[]  bOutMin=[]  bOutMax=[]  cOutMin=[]  cOutMax=[]  KbOutMin=[]  KbOutMax=[]  KtOutMin=[]  KtOutMax=[]  IntegratorOutMin=[]  IntegratorOutMax=[]  FilterOutMin=[]  FilterOutMax=[]  SumOutMin=[]  SumOutMax=[]  Sum1OutMin=[]  Sum1OutMax=[]  Sum2OutMin=[]  Sum2OutMax=[]  Sum3OutMin=[]  Sum3OutMax=[]  SumI1OutMin=[]  SumI1OutMax=[]  SumI2OutMin=[]  SumI2OutMax=[]  SumI3OutMin=[]  SumI3OutMax=[]  SumDOutMin=[]  SumDOutMax=[]  SaturationOutMin=[]  SaturationOutMax=[]  IntegratorContinuousStateAttributes=''  IntegratorStateMustResolveToSignalObject=off  IntegratorRTWStateStorageClass=Auto  FilterContinuousStateAttributes=''  FilterStateMustResolveToSignalObject=off  FilterRTWStateStorageClass=Auto  DifferentiatorICPrevScaledInput=0  DifferentiatorOutMin=[]  DifferentiatorOutMax=[]  FilterDiffOutCoefMin=[]  FilterDiffOutCoefMax=[]  SumDenOutMin=[]  SumDenOutMax=[]  SumNumOutMin=[]  SumNumOutMax=[]  ReciprocalOutMin=[]  ReciprocalOutMax=[]  DivideOutMin=[]  DivideOutMax=[]  TunerSelectOption=Transfer Function Based (PID Tuner App)
  cfblk4 : simulink/Discrete/Transfer Fcn Lead or Lag  PoleZ=0.95  ZeroZ=0.75  ICPrevOutput=0.0  ICPrevInput=0.0  DoSatur=off
      settings: SourceProductName=Simulink  SourceProductBaseCode=SL
  cfblk5 : DiscreteIntegrator  SampleTime=-1  OutDataTypeStr=double  ICPrevOutput=DiscIntNeverNeededParam  ICPrevScaledInput=DiscIntNeverNeededParam
  cfblk6 : simulink/Discrete/Difference  ICPrevInput=0.0  OutMin=[]  OutMax=[]  OutDataTypeStr=double  OutputDataTypeScalingMode=double  OutDataType=fixdt(1, 16)  OutScaling=2^-10  DoSatur=off
  cfblk7 : Delay  DelayLengthSource=Input port
      settings: InputPortMap=u0,p1
  cyemi_{1073..1080} (8 alike) : DataTypeConversion  OutDataTypeStr=double
  cfblk2 : Outport
  wires:
  cfblk5/1 -> cfblk2/1
  cyemi_1073/1 -> cfblk10/1
  cfblk4/1 -> cyemi_1073/1
  cyemi_1074/1 -> cfblk3/1
  cfblk10/1 -> cyemi_1074/1
  cyemi_1075/1 -> cfblk3/2
  cfblk9/1 -> cyemi_1075/1
  cyemi_1076/1 -> cfblk4/1
  cfblk3/1 -> cyemi_1076/1
  cyemi_1077/1 -> cfblk5/1
  cfblk7/1 -> cyemi_1077/1
  cyemi_1078/1 -> cfblk6/1
  cfblk1/1 -> cyemi_1078/1
  cyemi_1079/1 -> cfblk7/1
  cfblk6/1 -> cyemi_1079/1
  cyemi_1080/1 -> cfblk7/2
  cfblk8/1 -> cyemi_1080/1

== system sampleModel7126_pp/cfblk288 ==
  cfblk1 : Inport
  cfblk13 : Inport  Port=2
  Action Port : ActionPort  ActionType=else
  cfblk10 : simulink/Discrete/Tapped Delay  vinit=0.0  samptime=-1  NumDelays=1  DelayOrder=Oldest  includeCurrent=off
  cfblk11 : simulink/Discrete/Transfer Fcn First Order  PoleZ=0.95  ICPrevOutput=0.0  DoSatur=off
      settings: SourceProductName=Simulink
  cfblk12 : DiscreteStateSpace  SampleTime=-1
  cfblk3 : simulink/Continuous/PID Controller  Controller=PID  TimeDomain=Discrete-time  SampleTime=-1  IntegratorMethod=Forward Euler  FilterMethod=Forward Euler  Form=Parallel  UseFilter=on  ControllerParametersSource=internal  P=1  I=1  D=0  N=100  InitialConditionSource=internal  InitialConditionForIntegrator=0  InitialConditionForFilter=0  ExternalReset=none  LimitOutput=off  UpperSaturationLimit=inf  LowerSaturationLimit=-inf  LinearizeAsGain=off  AntiWindupMode=none  Kb=1  TrackingMode=off  Kt=1  PParamMin=[]  PParamMax=[]  IParamMin=[]  IParamMax=[]  DParamMin=[]  DParamMax=[]  NParamMin=[]  NParamMax=[]  KbParamMin=[]  KbParamMax=[]  KtParamMin=[]  KtParamMax=[]  POutMin=[]  POutMax=[]  IOutMin=[]  IOutMax=[]  DOutMin=[]  DOutMax=[]  NOutMin=[]  NOutMax=[]  KbOutMin=[]  KbOutMax=[]  KtOutMin=[]  KtOutMax=[]  IntegratorOutMin=[]  IntegratorOutMax=[]  FilterOutMin=[]  FilterOutMax=[]  SumOutMin=[]  SumOutMax=[]  SumI1OutMin=[]  SumI1OutMax=[]  SumI2OutMin=[]  SumI2OutMax=[]  SumI3OutMin=[]  SumI3OutMax=[]  SumDOutMin=[]  SumDOutMax=[]  SaturationOutMin=[]  SaturationOutMax=[]  IntegratorContinuousStateAttributes=''  IntegratorStateMustResolveToSignalObject=off  IntegratorRTWStateStorageClass=Auto  FilterContinuousStateAttributes=''  FilterStateMustResolveToSignalObject=off  FilterRTWStateStorageClass=Auto  DifferentiatorICPrevScaledInput=0  DifferentiatorOutMin=[]  DifferentiatorOutMax=[]  FilterDiffOutCoefMin=[]  FilterDiffOutCoefMax=[]  SumDenOutMin=[]  SumDenOutMax=[]  SumNumOutMin=[]  SumNumOutMax=[]  ReciprocalOutMin=[]  ReciprocalOutMax=[]  DivideOutMin=[]  DivideOutMax=[]  TunerSelectOption=Transfer Function Based (PID Tuner App)
  cfblk4 : UnitDelay  SampleTime=-1
  cfblk5 : DiscreteFir
  cfblk6 : Delay  ShowEnablePort=on
      settings: InputPortMap=u0,e6
  cfblk7 : simulink/Discrete/Transfer Fcn First Order  PoleZ=0.95  ICPrevOutput=0.0  DoSatur=off
      settings: SourceProductName=Simulink
  cfblk8 : simulink/Continuous/PID Controller  Controller=PID  TimeDomain=Discrete-time  SampleTime=-1  IntegratorMethod=Forward Euler  FilterMethod=Forward Euler  Form=Parallel  UseFilter=on  ControllerParametersSource=internal  P=1  I=1  D=0  N=100  InitialConditionSource=internal  InitialConditionForIntegrator=0  InitialConditionForFilter=0  ExternalReset=none  LimitOutput=off  UpperSaturationLimit=inf  LowerSaturationLimit=-inf  LinearizeAsGain=off  AntiWindupMode=none  Kb=1  TrackingMode=off  Kt=1  PParamMin=[]  PParamMax=[]  IParamMin=[]  IParamMax=[]  DParamMin=[]  DParamMax=[]  NParamMin=[]  NParamMax=[]  KbParamMin=[]  KbParamMax=[]  KtParamMin=[]  KtParamMax=[]  POutMin=[]  POutMax=[]  IOutMin=[]  IOutMax=[]  DOutMin=[]  DOutMax=[]  NOutMin=[]  NOutMax=[]  KbOutMin=[]  KbOutMax=[]  KtOutMin=[]  KtOutMax=[]  IntegratorOutMin=[]  IntegratorOutMax=[]  FilterOutMin=[]  FilterOutMax=[]  SumOutMin=[]  SumOutMax=[]  SumI1OutMin=[]  SumI1OutMax=[]  SumI2OutMin=[]  SumI2OutMax=[]  SumI3OutMin=[]  SumI3OutMax=[]  SumDOutMin=[]  SumDOutMax=[]  SaturationOutMin=[]  SaturationOutMax=[]  IntegratorContinuousStateAttributes=''  IntegratorStateMustResolveToSignalObject=off  IntegratorRTWStateStorageClass=Auto  FilterContinuousStateAttributes=''  FilterStateMustResolveToSignalObject=off  FilterRTWStateStorageClass=Auto  DifferentiatorICPrevScaledInput=0  DifferentiatorOutMin=[]  DifferentiatorOutMax=[]  FilterDiffOutCoefMin=[]  FilterDiffOutCoefMax=[]  SumDenOutMin=[]  SumDenOutMax=[]  SumNumOutMin=[]  SumNumOutMax=[]  ReciprocalOutMin=[]  ReciprocalOutMax=[]  DivideOutMin=[]  DivideOutMax=[]  TunerSelectOption=Transfer Function Based (PID Tuner App)
  cfblk9 : DiscreteTransferFcn
  cyemi_{1083..1093} (11 alike) : DataTypeConversion  OutDataTypeStr=double
  cfblk2 : Outport
  wires:
  cfblk12/1 -> cfblk2/1
  cyemi_1083/1 -> cfblk10/1
  cfblk8/1 -> cyemi_1083/1
  cyemi_1084/1 -> cfblk11/1
  cfblk4/1 -> cyemi_1084/1
  cyemi_1085/1 -> cfblk12/1
  cfblk11/1 -> cyemi_1085/1
  cyemi_1086/1 -> cfblk3/1
  cfblk6/1 -> cyemi_1086/1
  cyemi_1087/1 -> cfblk4/1
  cfblk7/1 -> cyemi_1087/1
  cyemi_1088/1 -> cfblk5/1
  cfblk3/1 -> cyemi_1088/1
  cyemi_1089/1 -> cfblk6/1
  cfblk1/1 -> cyemi_1089/1
  cyemi_1090/1 -> cfblk6/2
  cfblk13/1 -> cyemi_1090/1
  cyemi_1091/1 -> cfblk7/1
  cfblk9/1 -> cyemi_1091/1
  cyemi_1092/1 -> cfblk8/1
  cfblk5/1 -> cyemi_1092/1
  cyemi_1093/1 -> cfblk9/1
  cfblk10/1 -> cyemi_1093/1

== system sampleModel7126_pp/cfblk289 ==
  cfblk1 : Inport
  Action Port : ActionPort  ActionType=then
  cfblk10 : Subsystem  TreatAsAtomicUnit=on
  cfblk11 : Delay
  cfblk12 : Delay
  cfblk3 : simulink/Discrete/Transfer Fcn First Order  PoleZ=0.95  ICPrevOutput=0.0  DoSatur=off
      settings: SourceProductName=Simulink
  cfblk4 : DiscreteStateSpace  SampleTime=-1
  cfblk5 : simulink/Discrete/Transfer Fcn Real Zero  ZeroZ=0.75  ICPrevInput=0.0  DoSatur=off
      settings: SourceProductName=Simulink  SourceProductBaseCode=SL
  cfblk6 : DiscreteZeroPole  Poles=[0 0.5]  Gain=1  SampleTime=-1
  cfblk7 : If  SampleTime=1
  cfblk9 : Subsystem  TreatAsAtomicUnit=on
  cyemi_{1095..1096,1108..1116} (11 alike) : DataTypeConversion  OutDataTypeStr=double
  cfblk2 : Outport
  cfblk8 : Outport  Port=2
  wires:
  cfblk4/1 -> cyemi_1114/1, cyemi_1115/1, cyemi_1116/1
  cfblk6/1 -> cfblk2/1
  cfblk1/1 -> cfblk8/1, cyemi_1110/1
  cfblk7/1 -> cfblk9/Action
  cfblk7/2 -> cfblk10/Action
  cyemi_1095/1 -> cfblk10/1(cfblk1)
  cfblk3/1 -> cyemi_1095/1
  cyemi_1096/1 -> cfblk10/2(cfblk12)
  cfblk11/1 -> cyemi_1096/1
  cyemi_1108/1 -> cfblk11/1
  cfblk5/1 -> cyemi_1108/1
  cyemi_1109/1 -> cfblk12/1
  cfblk9/2(cfblk17) -> cyemi_1109/1
  cyemi_1110/1 -> cfblk3/1
  cyemi_1111/1 -> cfblk4/1
  cfblk12/1 -> cyemi_1111/1
  cyemi_1112/1 -> cfblk5/1
  cfblk10/1(cfblk2) -> cyemi_1112/1
  cyemi_1113/1 -> cfblk6/1
  cfblk9/1(cfblk2) -> cyemi_1113/1
  cyemi_1114/1 -> cfblk7/1
  cyemi_1115/1 -> cfblk9/1(cfblk1)
  cyemi_1116/1 -> cfblk9/2(cfblk16)

== system sampleModel7126_pp/cfblk290 ==
  cfblk1 : Inport
  cfblk10 : Inport  Port=2
  cfblk11 : Inport  Port=3
  cfblk12 : Inport  Port=4
  Action Port : ActionPort  ActionType=else
  cfblk3 : DiscreteTransferFcn
  cfblk4 : simulink/Discrete/Transfer Fcn Real Zero  ZeroZ=0.75  ICPrevInput=0.0  DoSatur=off
      settings: SourceProductName=Simulink  SourceProductBaseCode=SL
  cfblk5 : DiscreteFilter
  cfblk6 : simulink/Continuous/PID Controller (2DOF)  Controller=PID  TimeDomain=Discrete-time  SampleTime=-1  IntegratorMethod=Forward Euler  FilterMethod=Forward Euler  Form=Parallel  UseFilter=on  ControllerParametersSource=internal  P=1  I=1  D=0  N=100  b=1  c=1  InitialConditionSource=internal  InitialConditionForIntegrator=0  InitialConditionForFilter=0  ExternalReset=none  LimitOutput=off  UpperSaturationLimit=inf  LowerSaturationLimit=-inf  LinearizeAsGain=off  AntiWindupMode=none  Kb=1  TrackingMode=off  Kt=1  PParamMin=[]  PParamMax=[]  IParamMin=[]  IParamMax=[]  DParamMin=[]  DParamMax=[]  NParamMin=[]  NParamMax=[]  bParamMin=[]  bParamMax=[]  cParamMin=[]  cParamMax=[]  KbParamMin=[]  KbParamMax=[]  KtParamMin=[]  KtParamMax=[]  POutMin=[]  POutMax=[]  IOutMin=[]  IOutMax=[]  DOutMin=[]  DOutMax=[]  NOutMin=[]  NOutMax=[]  bOutMin=[]  bOutMax=[]  cOutMin=[]  cOutMax=[]  KbOutMin=[]  KbOutMax=[]  KtOutMin=[]  KtOutMax=[]  IntegratorOutMin=[]  IntegratorOutMax=[]  FilterOutMin=[]  FilterOutMax=[]  SumOutMin=[]  SumOutMax=[]  Sum1OutMin=[]  Sum1OutMax=[]  Sum2OutMin=[]  Sum2OutMax=[]  Sum3OutMin=[]  Sum3OutMax=[]  SumI1OutMin=[]  SumI1OutMax=[]  SumI2OutMin=[]  SumI2OutMax=[]  SumI3OutMin=[]  SumI3OutMax=[]  SumDOutMin=[]  SumDOutMax=[]  SaturationOutMin=[]  SaturationOutMax=[]  IntegratorContinuousStateAttributes=''  IntegratorStateMustResolveToSignalObject=off  IntegratorRTWStateStorageClass=Auto  FilterContinuousStateAttributes=''  FilterStateMustResolveToSignalObject=off  FilterRTWStateStorageClass=Auto  DifferentiatorICPrevScaledInput=0  DifferentiatorOutMin=[]  DifferentiatorOutMax=[]  FilterDiffOutCoefMin=[]  FilterDiffOutCoefMax=[]  SumDenOutMin=[]  SumDenOutMax=[]  SumNumOutMin=[]  SumNumOutMax=[]  ReciprocalOutMin=[]  ReciprocalOutMax=[]  DivideOutMin=[]  DivideOutMax=[]  TunerSelectOption=Transfer Function Based (PID Tuner App)
  cfblk7 : DiscreteFilter
  cfblk8 : Delay
  cfblk9 : DiscreteStateSpace  SampleTime=-1
  cyemi_{1138..1140,1142..1145} (7 alike) : DataTypeConversion  OutDataTypeStr=double
  cyemi_1141 : DataTypeConversion  OutDataTypeStr=uint8
  cfblk2 : Outport
  cfblk13 : Outport  Port=2
  cfblk14 : Outport  Port=3
  cfblk15 : Outport  Port=4
  cfblk16 : Outport  Port=5
  wires:
  cfblk1/1 -> cfblk15/1
  cfblk7/1 -> cfblk14/1
  cfblk6/1 -> cfblk2/1, cfblk16/1
  cfblk3/1 -> cfblk13/1
  cfblk4/1 -> cyemi_1138/1, cyemi_1142/1
  cyemi_1138/1 -> cfblk3/1
  cyemi_1139/1 -> cfblk4/1
  cfblk5/1 -> cyemi_1139/1
  cyemi_1140/1 -> cfblk5/1
  cfblk9/1 -> cyemi_1140/1
  cyemi_1141/1 -> cfblk6/1
  cfblk10/1 -> cyemi_1141/1
  cyemi_1142/1 -> cfblk6/2
  cyemi_1143/1 -> cfblk7/1
  cfblk11/1 -> cyemi_1143/1
  cyemi_1144/1 -> cfblk8/1
  cfblk12/1 -> cyemi_1144/1
  cyemi_1145/1 -> cfblk9/1
  cfblk8/1 -> cyemi_1145/1

== system sampleModel7126_pp/cfblk291 ==
  cfblk1 : Inport
  Action Port : ActionPort  ActionType=then
  cfblk3 : DiscreteTransferFcn
  cfblk4 : Delay  ShowEnablePort=on
      settings: InputPortMap=u0,e6
  cfblk5 : DiscreteZeroPole  Poles=[0 0.5]  Gain=1  SampleTime=-1
  cfblk6 : Delay  ShowEnablePort=on
      settings: InputPortMap=u0,e6
  cfblk7 : DiscreteFilter
  cyemi_{1147..1153} (7 alike) : DataTypeConversion  OutDataTypeStr=double
  cfblk2 : Outport
  cfblk8 : Outport  Port=2
  wires:
  cfblk6/1 -> cfblk2/1
  cfblk1/1 -> cfblk8/1, cyemi_1147/1, cyemi_1149/1, cyemi_1150/1
  cyemi_1147/1 -> cfblk3/1
  cyemi_1148/1 -> cfblk4/1
  cfblk3/1 -> cyemi_1148/1
  cyemi_1149/1 -> cfblk4/2
  cyemi_1150/1 -> cfblk5/1
  cyemi_1151/1 -> cfblk6/1
  cfblk7/1 -> cyemi_1151/1
  cyemi_1152/1 -> cfblk6/2
  cfblk4/1 -> cyemi_1152/1
  cyemi_1153/1 -> cfblk7/1
  cfblk5/1 -> cyemi_1153/1

== system sampleModel7126_pp/cfblk292 ==
  cfblk1 : Inport
  cfblk11 : Inport  Port=2
  Action Port : ActionPort  ActionType=else
  cfblk10 : If  SampleTime=1
  cfblk14 : Subsystem  TreatAsAtomicUnit=on
  cfblk15 : Subsystem  TreatAsAtomicUnit=on
  cfblk16 : Delay
  cfblk17 : Delay
  cfblk3 : UnitDelay  SampleTime=-1
  cfblk4 : Delay  ShowEnablePort=on
      settings: InputPortMap=u0,e6
  cfblk5 : simulink/Discrete/Transfer Fcn Lead or Lag  PoleZ=0.95  ZeroZ=0.75  ICPrevOutput=0.0  ICPrevInput=0.0  DoSatur=off
      settings: SourceProductName=Simulink  SourceProductBaseCode=SL
  cfblk6 : simulink/Discrete/Tapped Delay  vinit=0.0  samptime=-1  NumDelays=1  DelayOrder=Oldest  includeCurrent=off
  cfblk7 : simulink/Continuous/PID Controller  Controller=PID  TimeDomain=Discrete-time  SampleTime=-1  IntegratorMethod=Forward Euler  FilterMethod=Forward Euler  Form=Parallel  UseFilter=on  ControllerParametersSource=internal  P=1  I=1  D=0  N=100  InitialConditionSource=internal  InitialConditionForIntegrator=0  InitialConditionForFilter=0  ExternalReset=none  LimitOutput=off  UpperSaturationLimit=inf  LowerSaturationLimit=-inf  LinearizeAsGain=off  AntiWindupMode=none  Kb=1  TrackingMode=off  Kt=1  PParamMin=[]  PParamMax=[]  IParamMin=[]  IParamMax=[]  DParamMin=[]  DParamMax=[]  NParamMin=[]  NParamMax=[]  KbParamMin=[]  KbParamMax=[]  KtParamMin=[]  KtParamMax=[]  POutMin=[]  POutMax=[]  IOutMin=[]  IOutMax=[]  DOutMin=[]  DOutMax=[]  NOutMin=[]  NOutMax=[]  KbOutMin=[]  KbOutMax=[]  KtOutMin=[]  KtOutMax=[]  IntegratorOutMin=[]  IntegratorOutMax=[]  FilterOutMin=[]  FilterOutMax=[]  SumOutMin=[]  SumOutMax=[]  SumI1OutMin=[]  SumI1OutMax=[]  SumI2OutMin=[]  SumI2OutMax=[]  SumI3OutMin=[]  SumI3OutMax=[]  SumDOutMin=[]  SumDOutMax=[]  SaturationOutMin=[]  SaturationOutMax=[]  IntegratorContinuousStateAttributes=''  IntegratorStateMustResolveToSignalObject=off  IntegratorRTWStateStorageClass=Auto  FilterContinuousStateAttributes=''  FilterStateMustResolveToSignalObject=off  FilterRTWStateStorageClass=Auto  DifferentiatorICPrevScaledInput=0  DifferentiatorOutMin=[]  DifferentiatorOutMax=[]  FilterDiffOutCoefMin=[]  FilterDiffOutCoefMax=[]  SumDenOutMin=[]  SumDenOutMax=[]  SumNumOutMin=[]  SumNumOutMax=[]  ReciprocalOutMin=[]  ReciprocalOutMax=[]  DivideOutMin=[]  DivideOutMax=[]  TunerSelectOption=Transfer Function Based (PID Tuner App)
  cfblk8 : simulink/Continuous/PID Controller  Controller=PID  TimeDomain=Discrete-time  SampleTime=-1  IntegratorMethod=Forward Euler  FilterMethod=Forward Euler  Form=Parallel  UseFilter=on  ControllerParametersSource=internal  P=1  I=1  D=0  N=100  InitialConditionSource=internal  InitialConditionForIntegrator=0  InitialConditionForFilter=0  ExternalReset=none  LimitOutput=off  UpperSaturationLimit=inf  LowerSaturationLimit=-inf  LinearizeAsGain=off  AntiWindupMode=none  Kb=1  TrackingMode=off  Kt=1  PParamMin=[]  PParamMax=[]  IParamMin=[]  IParamMax=[]  DParamMin=[]  DParamMax=[]  NParamMin=[]  NParamMax=[]  KbParamMin=[]  KbParamMax=[]  KtParamMin=[]  KtParamMax=[]  POutMin=[]  POutMax=[]  IOutMin=[]  IOutMax=[]  DOutMin=[]  DOutMax=[]  NOutMin=[]  NOutMax=[]  KbOutMin=[]  KbOutMax=[]  KtOutMin=[]  KtOutMax=[]  IntegratorOutMin=[]  IntegratorOutMax=[]  FilterOutMin=[]  FilterOutMax=[]  SumOutMin=[]  SumOutMax=[]  SumI1OutMin=[]  SumI1OutMax=[]  SumI2OutMin=[]  SumI2OutMax=[]  SumI3OutMin=[]  SumI3OutMax=[]  SumDOutMin=[]  SumDOutMax=[]  SaturationOutMin=[]  SaturationOutMax=[]  IntegratorContinuousStateAttributes=''  IntegratorStateMustResolveToSignalObject=off  IntegratorRTWStateStorageClass=Auto  FilterContinuousStateAttributes=''  FilterStateMustResolveToSignalObject=off  FilterRTWStateStorageClass=Auto  DifferentiatorICPrevScaledInput=0  DifferentiatorOutMin=[]  DifferentiatorOutMax=[]  FilterDiffOutCoefMin=[]  FilterDiffOutCoefMax=[]  SumDenOutMin=[]  SumDenOutMax=[]  SumNumOutMin=[]  SumNumOutMax=[]  ReciprocalOutMin=[]  ReciprocalOutMax=[]  DivideOutMin=[]  DivideOutMax=[]  TunerSelectOption=Transfer Function Based (PID Tuner App)
  cfblk9 : DiscreteTransferFcn
  cyemi_{1156..1157,1165..1168,1176..1185} (16 alike) : DataTypeConversion  OutDataTypeStr=double
  cfblk2 : Outport
  cfblk12 : Outport  Port=2
  cfblk13 : Outport  Port=3
  wires:
  cfblk8/1 -> cyemi_1176/1, cyemi_1178/1
  cfblk1/1 -> cyemi_1156/1, cyemi_1183/1
  cfblk3/1 -> cfblk12/1
  cfblk7/1 -> cfblk13/1
  cfblk15/1(cfblk2) -> cfblk2/1
  cfblk14/2(cfblk7) -> cyemi_1168/1, cyemi_1181/1
  cfblk10/1 -> cfblk14/Action
  cfblk10/2 -> cfblk15/Action
  cyemi_1156/1 -> cfblk10/1
  cyemi_1157/1 -> cfblk14/1(cfblk1)
  cfblk17/1 -> cyemi_1157/1
  cyemi_1165/1 -> cfblk15/1(cfblk1)
  cfblk14/1(cfblk2) -> cyemi_1165/1
  cyemi_1166/1 -> cfblk15/2(cfblk8)
  cfblk11/1 -> cyemi_1166/1
  cyemi_1167/1 -> cfblk15/3(cfblk9)
  cfblk16/1 -> cyemi_1167/1
  cyemi_1168/1 -> cfblk15/4(cfblk10)
  cyemi_1176/1 -> cfblk16/1
  cyemi_1177/1 -> cfblk17/1
  cfblk15/3(cfblk12) -> cyemi_1177/1
  cyemi_1178/1 -> cfblk3/1
  cyemi_1179/1 -> cfblk4/1
  cfblk5/1 -> cyemi_1179/1
  cyemi_1180/1 -> cfblk4/2
  cfblk9/1 -> cyemi_1180/1
  cyemi_1181/1 -> cfblk5/1
  cyemi_1182/1 -> cfblk6/1
  cfblk4/1 -> cyemi_1182/1
  cyemi_1183/1 -> cfblk7/1
  cyemi_1184/1 -> cfblk8/1
  cfblk6/1 -> cyemi_1184/1
  cyemi_1185/1 -> cfblk9/1
  cfblk15/2(cfblk11) -> cyemi_1185/1
